simulink model "clase19012021"  (R2020b)
settings: Solver=VariableStepAuto  StartTime=0.0  StopTime=50/100  RelTol=1e-3
libraries: commdigbbndcpm2 x1, commrandsrc3 x1
settings Model: Creator=fernando  LastModifiedBy=fernando

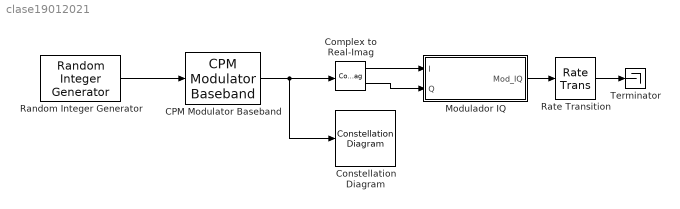
== system clase19012021 ==
  CPM Modulator Baseband : commdigbbndcpm2/CPM Modulator Baseband  Mnum=2  inputType=Bit  mappingType=Binary  modIdx=0.5  pulseShape=Rectangular  BT=0.3  mainLobePulseLength=1  rollOff=0.2  pulseLength=1  preHistory=1  phaseOffset=0  samplesPerSymbol=8  RateOptions=Allow multirate processing  outDataType=double
      settings: SourceProductBaseCode=CM
  Complex to Real-Imag : ComplexToRealImag
  Constellation Diagram : ConstellationDiagram
  Modulador IQ : Subsystem
  Random Integer Generator : commrandsrc3/Random Integer Generator  SetSize=2  SeedSource=Auto  Seed=0  SampleTime=1/500  SamplesPerFrame=1  OutputDataType=boolean  SimulateUsing=Interpreted execution
  Rate Transition : RateTransition  OutPortSampleTime=1/8e3/10
  Terminator : Terminator
  wires:
  Random Integer Generator/1 -> CPM Modulator Baseband/1
  CPM Modulator Baseband/1 -> Constellation Diagram/1, Complex to Real-Imag/1
  Complex to Real-Imag/1 -> Modulador IQ/1(I)
  Complex to Real-Imag/2 -> Modulador IQ/2(Q)
  Modulador IQ/1(Mod_IQ) -> Rate Transition/1
  Rate Transition/1 -> Terminator/1

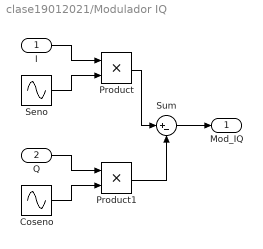
== system clase19012021/Modulador IQ ==
  I : Inport
  Q : Inport  Port=2
  Coseno : Sin  Frequency=2*pi*1e3  Phase=pi/2  SampleTime=0
  Product : Product
  Product1 : Product
  Seno : Sin  Frequency=2*pi*1e3  SampleTime=0
  Sum : Sum  Inputs=|+-
  Mod_IQ : Outport
  wires:
  Seno/1 -> Product/2
  I/1 -> Product/1
  Coseno/1 -> Product1/2
  Product1/1 -> Sum/2
  Sum/1 -> Mod_IQ/1
  Product/1 -> Sum/1
  Q/1 -> Product1/1
